simulink model "Pole_Placement_ohne_d"  (Simulink 7.5)
settings: Solver=ode45  StartTime=0.0  StopTime=10.0  RelTol=1e-3
undefined symbols (not defined in the file or in its folder): A, b, cT
settings Model: Creator=Mattse  LastModifiedBy=Mattse

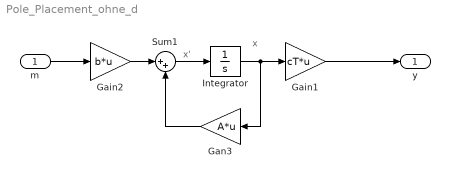
== system Pole_Placement_ohne_d ==
  note: x'
  note: x
  m : Inport  OutDataType=fixdt(1, 16)  OutScaling=2^0
  Gain1 : Gain  Gain=cT*u  ParameterDataType=fixdt(1, 16)  ParameterScaling=2^0  OutDataType=fixdt(1, 16)  OutScaling=2^0
  Gain2 : Gain  Gain=b*u  ParameterDataType=fixdt(1, 16)  ParameterScaling=2^0  OutDataType=fixdt(1, 16)  OutScaling=2^0
  Gan3 : Gain  Gain=A*u  ParameterDataType=fixdt(1, 16)  ParameterScaling=2^0  OutDataType=fixdt(1, 16)  OutScaling=2^0
  Integrator : Integrator
  Sum1 : Sum  Inputs=|++  OutDataType=fixdt(1, 16)  OutScaling=2^0
  y : Outport  OutDataType=fixdt(1, 16)  OutScaling=2^0
  wires:
  Integrator/1 -> Gain1/1, Gan3/1
  Sum1/1 -> Integrator/1
  m/1 -> Gain2/1
  Gain2/1 -> Sum1/1
  Gan3/1 -> Sum1/2
  Gain1/1 -> y/1
